simulink model "DroneNonLinearModel_v2"  (R2022b)
settings: Solver=VariableStepAuto  StartTime=0.0  StopTime=10.0  RelTol=1e-3
libraries: shared6dof x1
settings Model: Creator=bendr  LastModifiedBy=bendr

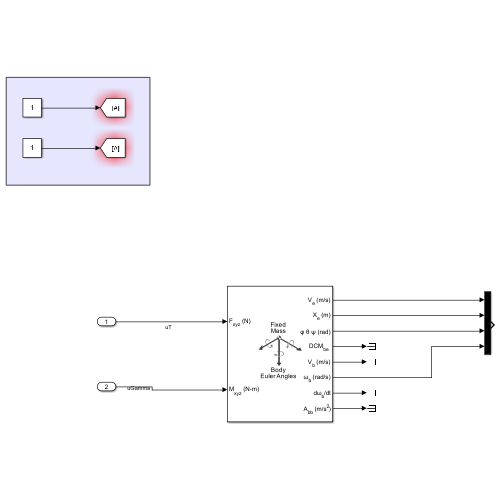
[thumbnail: Simulink's stored preview of the top-level diagram]
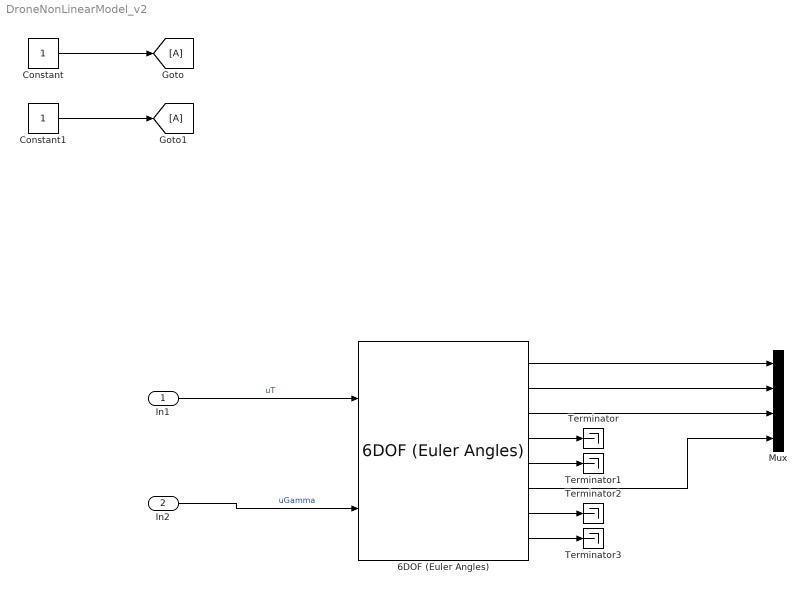
== system DroneNonLinearModel_v2 ==
  In1 : Inport
  In2 : Inport  Port=2
  6DOF (Euler Angles) : shared6dof/6DOF (Euler Angles)  units=Metric (MKS)  mtype=Fixed  rep=Euler Angles  xme_0=[0 0 0]  Vm_0=[0 0 0]  eul_0=[0 0 0]  pm_0=[0 0 0]  mass_0=1.0  mass_e=0.5  mass_f=2.0  inertia=eye(3)  inertia_e=eye(3)  inertia_f=2*eye(3)  k_quat=1.0  vre_flag=on  abi_flag=off  aMode=0  xme_statename={'Xe', 'Ye', 'Ze'}  Vm_statename={'U', 'v', 'w'}  eul_statename={'phi', 'theta', 'psi'}  quat_statename=''  pm_statename={'p', 'q', 'r'}  mass_statename=''
  Constant : Constant
  Constant1 : Constant
  Goto : Goto
  Goto1 : Goto
  Mux : Mux
  Terminator{,1..3} (4 alike) : Terminator
  wires:
  In1/1 -> 6DOF (Euler Angles)/1  "uT"
  In2/1 -> 6DOF (Euler Angles)/2  "uGamma"
  6DOF (Euler Angles)/4 -> Terminator/1
  6DOF (Euler Angles)/1 -> Mux/1
  6DOF (Euler Angles)/2 -> Mux/2
  6DOF (Euler Angles)/3 -> Mux/3
  6DOF (Euler Angles)/6 -> Mux/4
  6DOF (Euler Angles)/5 -> Terminator1/1
  6DOF (Euler Angles)/7 -> Terminator2/1
  6DOF (Euler Angles)/8 -> Terminator3/1
  Constant/1 -> Goto/1
  Constant1/1 -> Goto1/1
